simulink model "Problem6_21_BlockDiagram"  (R2020b)
settings: Solver=VariableStepAuto  StartTime=0.0  StopTime=10.0  RelTol=1e-3
values from neighbouring files (symbols this model uses):
  b = (b1 + b2)    (= 240)    [Problem6_14.m]    (also in Problem6_15.m; Problem6_20.m = 1608.49543864; Problem6_21.m = 1608.49543864; Problem6_23.m = 1608.49543864)
  d = 5*10^-2    (= 0.05)    [Problem6_21.m]
  k = m*w_n^2    (= 157913.670417)    [Problem6_20.m]    (also in Problem6_21.m; Problem6_23.m)
  m = 640    [Problem6_20.m]    (also in Problem6_21.m; Problem6_23.m)
  t_end = t_start + t_p    (= 4.6)    [Problem6_21.m]
  t_start = 1    [Problem6_21.m]
undefined symbols (not defined in the file or in its folder): x_init, y_init
settings Model: Creator=jonathanmoran  LastModifiedBy=jonathanmoran

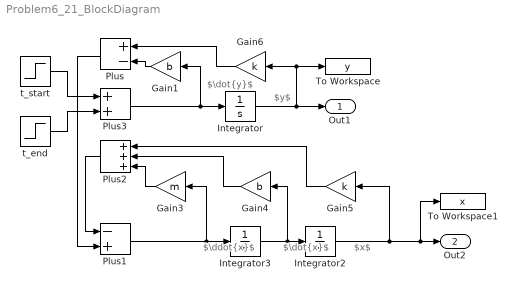
== system Problem6_21_BlockDiagram ==
  note: $x$
  note: $\dot{x}$
  note: $\dot{y}$
  note: $y$
  note: $\ddot{x}$
  Gain1 : Gain  Gain=b
  Gain3 : Gain  Gain=m
  Gain4 : Gain  Gain=b
  Gain5 : Gain  Gain=k
  Gain6 : Gain  Gain=k
  Integrator : Integrator  InitialCondition=y_init
  Integrator2 : Integrator  InitialCondition=x_init
  Integrator3 : Integrator  InitialCondition=x_init
  Plus : Sum  Inputs=+-
  Plus1 : Sum  Inputs=-+
  Plus2 : Sum  Inputs=+++
  Plus3 : Sum
  To Workspace : ToWorkspace  VariableName=y  SampleTime=-1
  To Workspace1 : ToWorkspace  VariableName=x  SampleTime=-1
  t_end : Step  Time=t_end  After=-d  SampleTime=0
  t_start : Step  Time=t_start  After=d  SampleTime=0
  Out1 : Outport  SignalName=y
  Out2 : Outport  Port=2  SignalName=x
  wires:
  Integrator3/1 -> Gain4/1, Integrator2/1
  Integrator/1 -> Gain6/1, To Workspace/1, Out1/1
  Plus1/1 -> Gain3/1, Integrator3/1
  Integrator2/1 -> To Workspace1/1, Out2/1, Gain5/1
  Gain3/1 -> Plus2/3
  Gain4/1 -> Plus2/2
  Gain5/1 -> Plus2/1
  Plus3/1 -> Gain1/1, Integrator/1
  Gain1/1 -> Plus/2
  Gain6/1 -> Plus/1
  Plus/1 -> Plus1/2
  Plus2/1 -> Plus1/1
  t_start/1 -> Plus3/1
  t_end/1 -> Plus3/2
